simulink model "testing_bits"  (R2022b)
settings: Solver=VariableStepAuto  StartTime=0.0  StopTime=0.2  MaxStep=1e-4  RelTol=1e-3
values from neighbouring files (symbols this model uses):
  f = 50    [DFIG_init1.m]    (also in DFIG_init3.m; DFIG_init4.m; DFIG_init5.m; DFIG_init6.m)
  Ts = 1/fsw/50    (= 5e-06)    [DFIG_init1.m]    (also in DFIG_init3.m; DFIG_init4.m; DFIG_init5.m; DFIG_init6.m)
  Vs = 690    [DFIG_init1.m]    (also in DFIG_init3.m; DFIG_init4.m; DFIG_init5.m; DFIG_init6.m)
libraries: spsPLL3phLib x3, spsCurrentMeasurementLib x1, spsGroundLib x1, spsThreePhaseProgrammableVoltageSourceLib x1, spsThreePhaseVIMeasurementLib x1, spsVoltageMeasurementLib x1, sps_lib x1
settings Model: Creator=Qingyuan  LastModifiedBy=Qingyuan

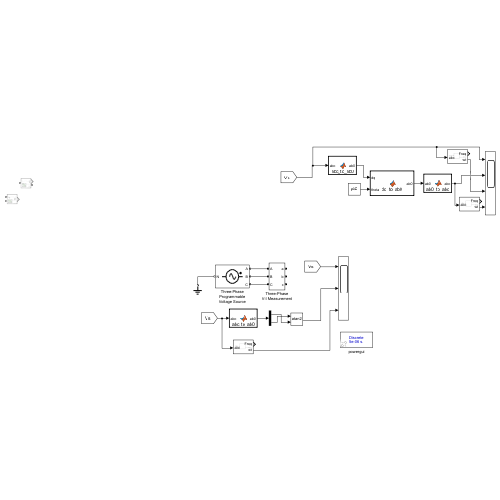
[thumbnail: Simulink's stored preview of the top-level diagram]
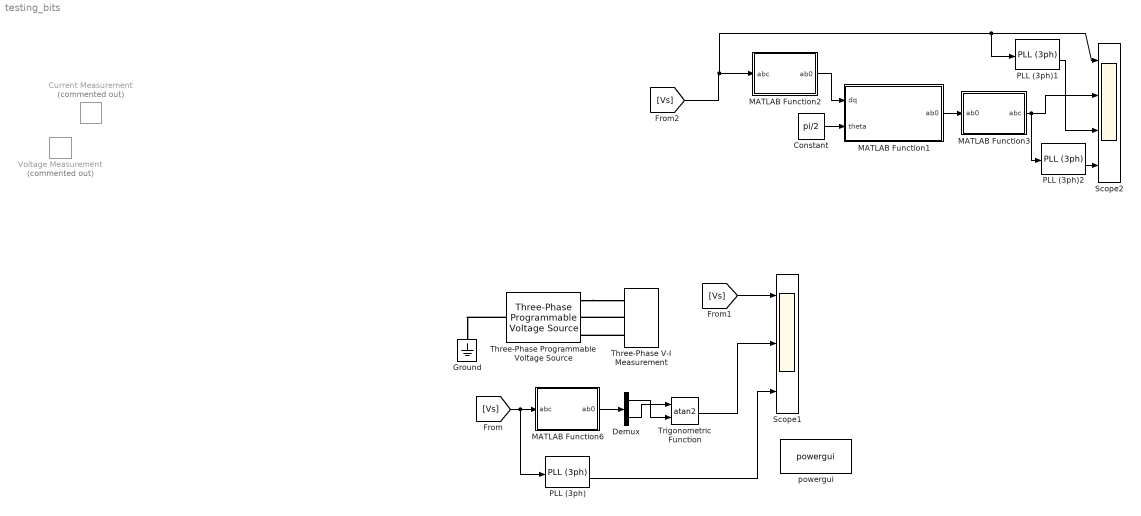
== system testing_bits ==
  Constant : Constant  Value=pi/2
  Current Measurement : spsCurrentMeasurementLib/Current Measurement  Commented=on  PhasorSimulation=off  OutputType=Complex  PSBequivalent=0
  Demux : Demux  Outputs=2
  Ground : spsGroundLib/Ground  LConnTagsString=a
  MATLAB Function1 : MATLAB Function  TreatAsAtomicUnit=on
  MATLAB Function2 : MATLAB Function  TreatAsAtomicUnit=on
  MATLAB Function3 : MATLAB Function  TreatAsAtomicUnit=on
  MATLAB Function6 : MATLAB Function  TreatAsAtomicUnit=on
  PLL (3ph) : spsPLL3phLib/PLL (3ph)  Fmin=45  Par_Init=[0, 50]  ParK=[180, 3200, 1]  TcD=1e-4  MaxRateChangeFreq=12  FilterCutOffFreq=25  Ts=0  AGC=on
  PLL (3ph)1 : spsPLL3phLib/PLL (3ph)  Fmin=45  Par_Init=[0, 50]  ParK=[180, 3200, 1]  TcD=1e-4  MaxRateChangeFreq=12  FilterCutOffFreq=25  Ts=0  AGC=on
  PLL (3ph)2 : spsPLL3phLib/PLL (3ph)  Fmin=45  Par_Init=[0, 50]  ParK=[180, 3200, 1]  TcD=1e-4  MaxRateChangeFreq=12  FilterCutOffFreq=25  Ts=0  AGC=on
  Scope1 : Scope  NumInputPorts=3
  Scope2 : Scope  NumInputPorts=4
  Three-Phase Programmable Voltage Source : spsThreePhaseProgrammableVoltageSourceLib/Three-Phase Programmable Voltage Source  PositiveSequence="[Vs  0 f]"  VariationEntity=None  VariationType=Table of time-amplitude pairs  VariationTypeAlt=Step  VariationStep=0.5  VariationRate=10  VariationMagnitude=0.3  VariationFrequency=2  VariationTiming=[1 2]  VariationPhaseA=off  Amplitudes=[1 0.8 1.2 1.0]  TimeValues=[0 0.1 0.15 0.2]  HarmonicGeneration=off  HarmonicA=[3 0.2 -25 0]  HarmonicB=[2 0.15 35 2]  Timing="[0.05  3]"  BusType=swing  Pref=0  Qref=0  Qmin=-inf  Qmax=inf
  Three-Phase V-I Measurement : spsThreePhaseVIMeasurementLib/Three-Phase V-I Measurement  VoltageMeasurement=phase-to-ground  SetLabelV=on  LabelV=Vs  Vpu=off  VpuLL=off  CurrentMeasurement=yes  SetLabelI=on  LabelI=Is  Ipu=off  Pbase=100e6  Vbase=500e3  OutputType=Complex  PhasorSimulation=off  PSBequivalent=0
  Trigonometric Function : Trigonometry  Operator=atan2
  Voltage Measurement : spsVoltageMeasurementLib/Voltage Measurement  Commented=on  PhasorSimulation=off  OutputType=Complex  PSBequivalent=0
  powergui : sps_lib/powergui  Priority=1  SimulationMode=Discrete  SampleTime=Ts  frequency=60  Iterations=50  frequencyindice=50  Pbase=100e6  ErrMax=1e-4  UnitsV=kV  UnitsW=MW  buscounter=0  FunctionMessages=off  echomessages=off  EnableUseOfTLC=off  CurrentSourceSwitches=off  DisableSnubberDevices=off  DisableRonSwitches=off  DisableVfSwitches=off  DisplayEquations=off  AutomaticDiscreteSolvers=off  SolverType=Tustin/Backward Euler (TBE)  Interpol=off  ExternalGateDelay=off  methode=off  Ts=100  x0status=blocks  SPID=on  SwTol=0  HookPort=off  NonlinearTolerance=1e-4  nMaxIteration=100  ContinueOnMaxIteration=off  RestoreLinks=warning  ResistiveCurrentMeasurement=off  Frange=[0:2:500]  Ylog=off  Xlog=on  ShowGrid=off  save=off  variable=ZData  structure=0  ZoomFFT=off  StartTime=0.0  cycles=1  DisplayStyle=1  fundamental=60  FreqAxis=off  MaxFrequency=1000  frequencyindicesteady=1  RmsSteady=1  display=off
  wires:
  MATLAB Function1/1(ab0) -> MATLAB Function3/1(ab0)
  Constant/1 -> MATLAB Function1/2(theta)
  [Vs] -> PLL (3ph)/1, MATLAB Function6/1(abc)
  Demux/2 -> Trigonometric Function/1
  Demux/1 -> Trigonometric Function/2
  MATLAB Function6/1(ab0) -> Demux/1
  Trigonometric Function/1 -> Scope1/2
  PLL (3ph)/2 -> Scope1/3
  [Vs] -> Scope1/1
  [Vs] -> PLL (3ph)1/1, Scope2/1, MATLAB Function2/1(abc)
  MATLAB Function2/1(ab0) -> MATLAB Function1/1(dq)
  MATLAB Function3/1(abc) -> PLL (3ph)2/1, Scope2/2
  PLL (3ph)1/2 -> Scope2/3
  PLL (3ph)2/2 -> Scope2/4
  connections:
  Three-Phase V-I Measurement/LConn2 -- Three-Phase Programmable Voltage Source/RConn2
  Three-Phase V-I Measurement/LConn3 -- Three-Phase Programmable Voltage Source/RConn3
  Three-Phase Programmable Voltage Source/LConn1 -- Ground/LConn1
  Three-Phase Programmable Voltage Source/RConn1 -- Three-Phase V-I Measurement/LConn1

== matlab function testing_bits/MATLAB Function3 ==
  data: ab0 input; abc output
function abc = ab0_to_abc(ab0)
abc = zeros(3,1);
abc(1) = ab0(1);
abc(2) = -1/2 * ab0(1) + sqrt(3)/2 * ab0(2);
abc(3) = -1/2 * ab0(1) - sqrt(3)/2 * ab0(2);
end

== matlab function testing_bits/MATLAB Function6 ==
  data: abc input; ab0 output
function ab0 = abc_to_ab0(abc)
ab0 = zeros(2,1);
ab0(1) = 2/3 * (abc(1) - abc(2)/2 - abc(3)/2);
ab0(2) = 2/3 * ( (sqrt(3)/2)*abc(2) - (sqrt(3)/2)*abc(3));
end

== matlab function testing_bits/MATLAB Function2 ==
  data: abc input; ab0 output
function ab0 = abc_to_ab0(abc)
ab0 = zeros(2,1);
ab0(1) = 2/3 * (abc(1) - abc(2)/2 - abc(3)/2);
ab0(2) = 2/3 * ( (sqrt(3)/2)*abc(2) - (sqrt(3)/2)*abc(3));
end

== matlab function testing_bits/MATLAB Function1 ==
  data: dq input; ab0 output; theta input
function ab0 = dq_to_ab0(dq, theta)
ab0 = zeros(2,1);
ab0(1) = dq(1) * cos(theta) - dq(2) * sin(theta);
ab0(2) = dq(1) * sin(theta) + dq(2) * cos(theta);

end
